simulink model "servo_cherif"  (R2022b)
settings: Solver=VariableStepAuto  StartTime=0.0  StopTime=10.0  RelTol=1e-3
settings Model: Creator=castekcu  LastModifiedBy=castekcu

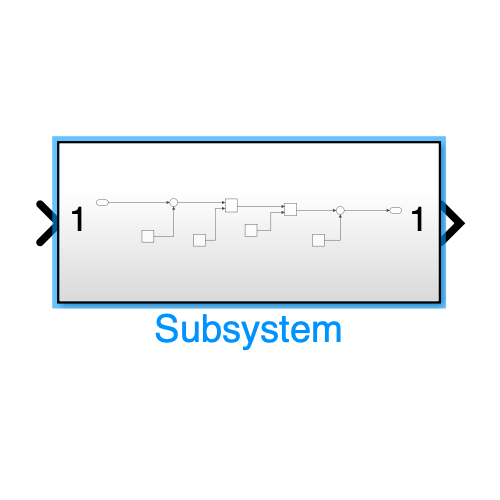
[thumbnail: Simulink's stored preview of the top-level diagram]
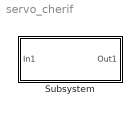
== system servo_cherif ==
  Subsystem : Subsystem

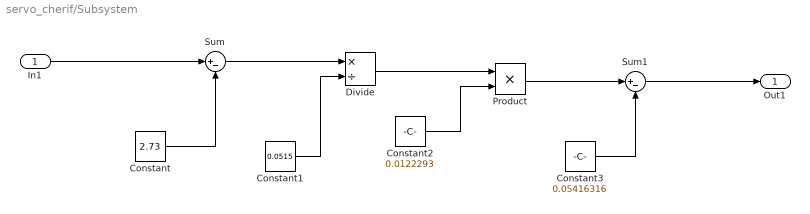
== system servo_cherif/Subsystem ==
  In1 : Inport
  Constant : Constant  Value=2.73
  Constant1 : Constant  Value=0.0515
  Constant2 : Constant  Value=0.0122293
  Constant3 : Constant  Value=0.05416316
  Divide : Product  Inputs=*/
  Product : Product
  Sum : Sum  Inputs=|+-
  Sum1 : Sum  Inputs=|+-
  Out1 : Outport
  wires:
  Constant/1 -> Sum/2
  Sum/1 -> Divide/1
  Constant1/1 -> Divide/2
  In1/1 -> Sum/1
  Divide/1 -> Product/1
  Constant2/1 -> Product/2
  Product/1 -> Sum1/1
  Constant3/1 -> Sum1/2
  Sum1/1 -> Out1/1
